simulink model "NavigationObserver_4"  (Simulink 8.3)
settings: configuration reference "mpc555rt_ref_debug_config" (kept outside this file)
values from neighbouring files (symbols this model uses):
  dt = 0.0192307692308    [newvars_4_25.mat]
  g = 32.174    [newvars_4_25.mat]
  P0_est_nav = [100 0 0 0 0 0 0 100 0 0 0 0 ... (36 elements, 6x6)]    [newvars_4_25.mat]
  Q_obs_nav = [0.001 0 0 0 0 0 0 0.001 0 0 0 0 ... (36 elements, 6x6)]    [newvars_4_25.mat]
  R_obs_nav = [0.001 0 0 0 0 0 0 0.001 0 0 0 0 ... (36 elements, 6x6)]    [newvars_4_25.mat]
  x0_est_nav = [0 0 200 0 0 0]    [newvars_4_25.mat]
libraries: simulink x1
(part 1 of 2)
settings Model: Creator=Rick Riley  LastModifiedBy=gagarcia
settings ConfigSet: SourceName=mpc555rt_ref_debug_config  SourceLocation=Base Workspace

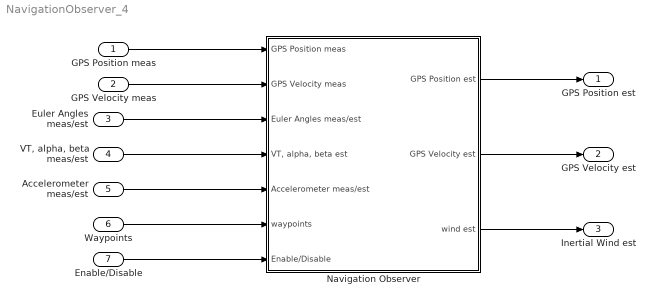
== system NavigationObserver_4 ==
  GPS Position meas : Inport  OutDataTypeStr=Bus: GPS_position_bus  SampleTime=dt
  GPS Velocity meas : Inport  Port=2  OutDataTypeStr=Bus: GPS_velocity_bus  SampleTime=dt  BusOutputAsStruct=on
  Euler Angles meas/est : Inport  Port=3  OutDataTypeStr=Bus: INS_angles_bus  SampleTime=dt
  "VT, alpha, beta meas/est" : Inport  Port=4  OutDataTypeStr=Bus: VT_A_B_bus  SampleTime=dt  BusOutputAsStruct=on
  Accelerometer meas/est : Inport  Port=5  OutDataTypeStr=Bus: Accelerometer
  Waypoints : Inport  Port=6  OutDataTypeStr=Bus: waypoint_bus  BusOutputAsStruct=on
  Enable/Disable : Inport  Port=7  OutDataTypeStr=boolean  SampleTime=dt
  Navigation Observer : Subsystem
  GPS Position est : Outport  OutDataTypeStr=Bus: GPS_position_bus  BusOutputAsStruct=on
  GPS Velocity est : Outport  Port=2  OutDataTypeStr=Bus: GPS_velocity_bus  BusOutputAsStruct=on
  Inertial Wind est : Outport  Port=3  OutDataTypeStr=Bus: Wind_bus  BusOutputAsStruct=on
  wires:
  Navigation Observer/3(wind est) -> Inertial Wind est/1
  GPS Position meas/1 -> Navigation Observer/1(GPS Position meas)
  GPS Velocity meas/1 -> Navigation Observer/2(GPS Velocity meas)
  Navigation Observer/1(GPS Position est) -> GPS Position est/1
  Navigation Observer/2(GPS Velocity est) -> GPS Velocity est/1
  Euler Angles meas/est/1 -> Navigation Observer/3(Euler Angles meas/est)
  "VT, alpha, beta meas/est"/1 -> Navigation Observer/4("VT, alpha, beta est")
  Accelerometer meas/est/1 -> Navigation Observer/5(Accelerometer meas/est)
  Waypoints/1 -> Navigation Observer/6(waypoints)
  Enable/Disable/1 -> Navigation Observer/7(Enable/Disable)

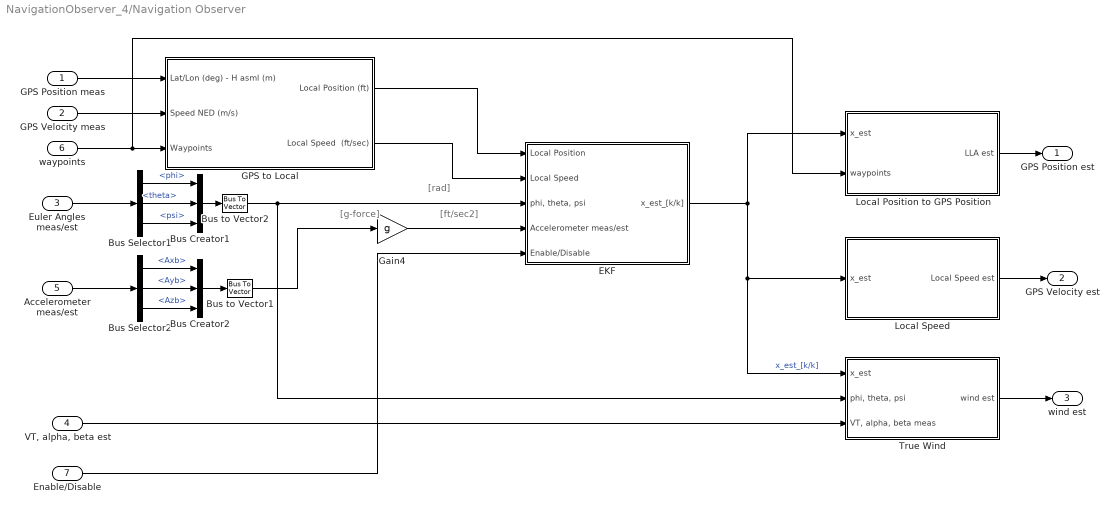
== system NavigationObserver_4/Navigation Observer ==
  note: [ft/sec2]
  note: [g-force]
  note: [rad]
  GPS Position meas : Inport  OutDataTypeStr=Bus: GPS_position_bus  SampleTime=dt
  GPS Velocity meas : Inport  Port=2  OutDataTypeStr=Bus: GPS_velocity_bus  SampleTime=dt  BusOutputAsStruct=on
  Euler Angles meas/est : Inport  Port=3  OutDataTypeStr=Bus: INS_angles_bus  SampleTime=dt
  "VT, alpha, beta est" : Inport  Port=4  OutDataTypeStr=Bus: VT_A_B_bus  SampleTime=dt  BusOutputAsStruct=on
  Accelerometer meas/est : Inport  Port=5  OutDataTypeStr=Bus: Accelerometer
  waypoints : Inport  Port=6  OutDataTypeStr=Bus: waypoint_bus
  Enable/Disable : Inport  Port=7  OutDataTypeStr=boolean  SampleTime=dt
  Bus Creator1 : BusCreator  Inputs=3  OutDataTypeStr=Bus: INS_angles_bus
  Bus Creator2 : BusCreator  Inputs=3  OutDataTypeStr=Bus: Accelerometer
  Bus Selector1 : BusSelector  OutputSignals=phi,theta,psi
  Bus Selector2 : BusSelector  OutputSignals=Axb,Ayb,Azb
  Bus to Vector1 : BusToVector
  Bus to Vector2 : BusToVector
  EKF : Subsystem
  GPS to Local : Subsystem
  Gain4 : Gain  Gain=g
  Local Position to GPS Position : Subsystem
  Local Speed : Subsystem
  True Wind : Subsystem
  GPS Position est : Outport  OutDataTypeStr=Bus: GPS_position_bus
  GPS Velocity est : Outport  Port=2
  wind est : Outport  Port=3
  wires:
  EKF/1(x_est_[k/k]) -> Local Position to GPS Position/1(x_est), Local Speed/1(x_est), True Wind/1(x_est)  "x_est_[k/k]"
  Euler Angles meas/est/1 -> Bus Selector1/1
  Accelerometer meas/est/1 -> Bus Selector2/1
  Bus to Vector1/1 -> Gain4/1
  GPS Position meas/1 -> GPS to Local/1(Lat/Lon (deg) - H asml (m))
  GPS Velocity meas/1 -> GPS to Local/2(Speed NED (m/s))
  waypoints/1 -> GPS to Local/3(Waypoints), Local Position to GPS Position/2(waypoints)
  GPS to Local/1(Local Position (ft)) -> EKF/1(Local Position)
  GPS to Local/2(Local Speed  (ft/sec)) -> EKF/2(Local Speed)
  Gain4/1 -> EKF/4(Accelerometer meas/est)
  Local Position to GPS Position/1(LLA est) -> GPS Position est/1
  Local Speed/1(Local Speed est) -> GPS Velocity est/1
  "VT, alpha, beta est"/1 -> True Wind/3("VT, alpha, beta meas")
  True Wind/1(wind est) -> wind est/1
  Bus to Vector2/1 -> EKF/3("phi, theta, psi"), True Wind/2("phi, theta, psi")
  Bus Selector1/1 -> Bus Creator1/1  "<phi>"
  Bus Selector1/2 -> Bus Creator1/2  "<theta>"
  Bus Selector1/3 -> Bus Creator1/3  "<psi>"
  Bus Creator1/1 -> Bus to Vector2/1
  Bus Selector2/1 -> Bus Creator2/1  "<Axb>"
  Bus Selector2/2 -> Bus Creator2/2  "<Ayb>"
  Bus Selector2/3 -> Bus Creator2/3  "<Azb>"
  Bus Creator2/1 -> Bus to Vector1/1
  Enable/Disable/1 -> EKF/5(Enable/Disable)

== system NavigationObserver_4/Navigation Observer/EKF ==
  Local Position : Inport
  Local Speed : Inport  Port=2
  "phi, theta, psi" : Inport  Port=3
  Accelerometer meas/est : Inport  Port=4
  Enable/Disable : Inport  Port=5  OutDataTypeStr=boolean  SampleTime=dt
  GPS rate correction : Subsystem
  Gain : Gain
  K[k] (navigation) : Subsystem
  Mux3 : Mux  Inputs=2
  Product : Product  RndMeth=Zero
  Product1 : Product  Multiplication=Matrix(*)  RndMeth=Zero
  Reshape1 : Reshape  OutputDimensionality=Column vector (2-D)
  Reshape2 : Reshape  OutputDimensionality=Column vector (2-D)
  Reshape3 : Reshape
  Subtract : Sum  Inputs=+-
  Subtract1 : Sum
  Unit Delay1 : UnitDelay  SampleTime=dt
  x_est_[0/0] : UnitDelay  InitialCondition=x0_est_nav  SampleTime=dt
  x_est_[k/k-1] : Subsystem
  y_[k] : Subsystem
  y_est_[k] : Subsystem
  x_est_[k/k] : Outport
  wires:
  y_[k]/1(y_[k]) -> Subtract/1, GPS rate correction/1(y_[k])
  Local Position/1 -> y_[k]/1(Local Position)
  x_est_[k/k-1]/1(x_est_[k/k-1]) -> y_est_[k]/1(x_est [k]), Reshape1/1
  Subtract1/1 -> Reshape3/1  "x_est_[k/k]"
  x_est_[0/0]/1 -> K[k] (navigation)/2(x_est_[k-1/k-1]), x_est_[k/k-1]/2(x_est_[k-1/k-1])  "x_est_[k-1/k-1]"
  Mux3/1 -> Unit Delay1/1  "u_[k]"
  Unit Delay1/1 -> K[k] (navigation)/1(u_[k-1]), x_est_[k/k-1]/1(u_[k-1])  "u_[k-1]"
  y_est_[k]/1(y_est_ [k]) -> Subtract/2
  Gain/1 -> Subtract1/1
  "phi, theta, psi"/1 -> Mux3/1
  Accelerometer meas/est/1 -> Mux3/2
  Local Speed/1 -> y_[k]/2(Local Speed)
  Product/1 -> Product1/1  "K_[k]"
  Product1/1 -> Gain/1
  Reshape1/1 -> Subtract1/2
  Reshape2/1 -> Product1/2
  Reshape3/1 -> x_est_[k/k]/1, x_est_[0/0]/1
  GPS rate correction/1(e_corrected_[k]) -> Reshape2/1
  Subtract/1 -> GPS rate correction/2(e_[k])
  K[k] (navigation)/1(K[k]) -> Product/1
  Enable/Disable/1 -> Product/2

== system NavigationObserver_4/Navigation Observer/GPS to Local ==
  Lat/Lon (deg) - H asml (m) : Inport
  Speed NED (m/s) : Inport  Port=2
  Waypoints : Inport  Port=3  OutDataTypeStr=Bus: waypoint_bus
  Bus Creator : BusCreator  Inputs=3  NonVirtualBus=on
  Bus Creator1 : BusCreator  Inputs=3  NonVirtualBus=on
  Bus Selector : BusSelector  OutputSignals=Altitude,Latitude,Longitude
  Bus Selector1 : BusSelector  OutputSignals=V_down,V_north,V_east
  Convert Lat/Lon/Alt to Flat Earth : MATLAB Function  TreatAsAtomicUnit=on
  Gain1 : Gain  Gain=-1
  Gain2 : Gain  Gain=1/.3048
  Gain3 : Gain  Gain=1/.3048
  Gain4 : Gain  Gain=1/.3048
  Local Position (ft) : Outport
  Local Speed  (ft/sec) : Outport  Port=2
  wires:
  Speed NED (m/s)/1 -> Bus Selector1/1
  Lat/Lon (deg) - H asml (m)/1 -> Bus Selector/1
  Bus Creator/1 -> Local Position (ft)/1
  Bus Selector1/2 -> Gain3/1  "<V_north>"
  Bus Selector1/1 -> Gain1/1  "<V_down>"
  Bus Selector1/3 -> Gain4/1  "<V_east>"
  Gain1/1 -> Gain2/1
  Gain4/1 -> Bus Creator1/3  "V_east"
  Gain3/1 -> Bus Creator1/2  "V_north"
  Gain2/1 -> Bus Creator1/1  "V_height"
  Bus Creator1/1 -> Local Speed  (ft/sec)/1
  Bus Selector/1 -> Convert Lat/Lon/Alt to Flat Earth/2(alt)  "<Altitude>"
  Bus Selector/2 -> Convert Lat/Lon/Alt to Flat Earth/3(lat)  "<Latitude>"
  Bus Selector/3 -> Convert Lat/Lon/Alt to Flat Earth/4(lon)  "<Longitude>"
  Convert Lat/Lon/Alt to Flat Earth/1(Height) -> Bus Creator/1
  Convert Lat/Lon/Alt to Flat Earth/2(North) -> Bus Creator/2
  Convert Lat/Lon/Alt to Flat Earth/3(East) -> Bus Creator/3
  Waypoints/1 -> Convert Lat/Lon/Alt to Flat Earth/1(wpts)

== system NavigationObserver_4/Navigation Observer/Local Position to GPS Position ==
  note: pn [ft]
  note: pe [ft]
  note: ph [ft]
  note: ve [ft/sec]
  note: vh [ft/sec]
  note: vn [ft/sec]
  x_est : Inport
  waypoints : Inport  Port=2  OutDataTypeStr=Bus: waypoint_bus
  Bus Creator : BusCreator  Inputs=3  OutDataTypeStr=Bus: GPS_position_bus  NonVirtualBus=on
  Convert Local Coordinates to LLA : MATLAB Function  TreatAsAtomicUnit=on
  Demux : Demux  Outputs=6
  Terminator : Terminator
  Terminator1 : Terminator
  Terminator2 : Terminator
  LLA est : Outport  OutDataTypeStr=Bus: GPS_position_bus
  wires:
  Convert Local Coordinates to LLA/3(Altitude) -> Bus Creator/3  "Altitude"
  Convert Local Coordinates to LLA/2(Longitude) -> Bus Creator/2  "Longitude"
  Convert Local Coordinates to LLA/1(Latitude) -> Bus Creator/1  "Latitude"
  x_est/1 -> Demux/1
  Bus Creator/1 -> LLA est/1
  Demux/4 -> Terminator/1
  Demux/5 -> Terminator1/1
  Demux/6 -> Terminator2/1
  Demux/1 -> Convert Local Coordinates to LLA/1(n)
  Demux/2 -> Convert Local Coordinates to LLA/2(e)
  Demux/3 -> Convert Local Coordinates to LLA/3(h)
  waypoints/1 -> Convert Local Coordinates to LLA/4(wpts)

== system NavigationObserver_4/Navigation Observer/Local Speed ==
  note: pn [ft]
  note: pe [ft]
  note: ph [ft]
  note: ve [ft/sec]
  note: vh [ft/sec]
  note: vn [ft/sec]
  x_est : Inport
  Bus Creator : BusCreator  Inputs=3  OutDataTypeStr=Bus: GPS_velocity_bus  NonVirtualBus=on
  Demux1 : Demux  Outputs=6
  Gain1 : Gain  Gain=0.3048
  Gain2 : Gain  Gain=0.3048
  Gain3 : Gain  Gain=-0.3048
  Terminator : Terminator
  Terminator1 : Terminator
  Terminator2 : Terminator
  Local Speed est : Outport
  wires:
  Bus Creator/1 -> Local Speed est/1
  Demux1/1 -> Terminator/1
  Demux1/2 -> Terminator1/1
  Demux1/3 -> Terminator2/1
  x_est/1 -> Demux1/1
  Gain2/1 -> Bus Creator/1  "V_north"
  Gain1/1 -> Bus Creator/2  "V_east"
  Gain3/1 -> Bus Creator/3  "V_down"
  Demux1/4 -> Gain2/1
  Demux1/5 -> Gain1/1
  Demux1/6 -> Gain3/1

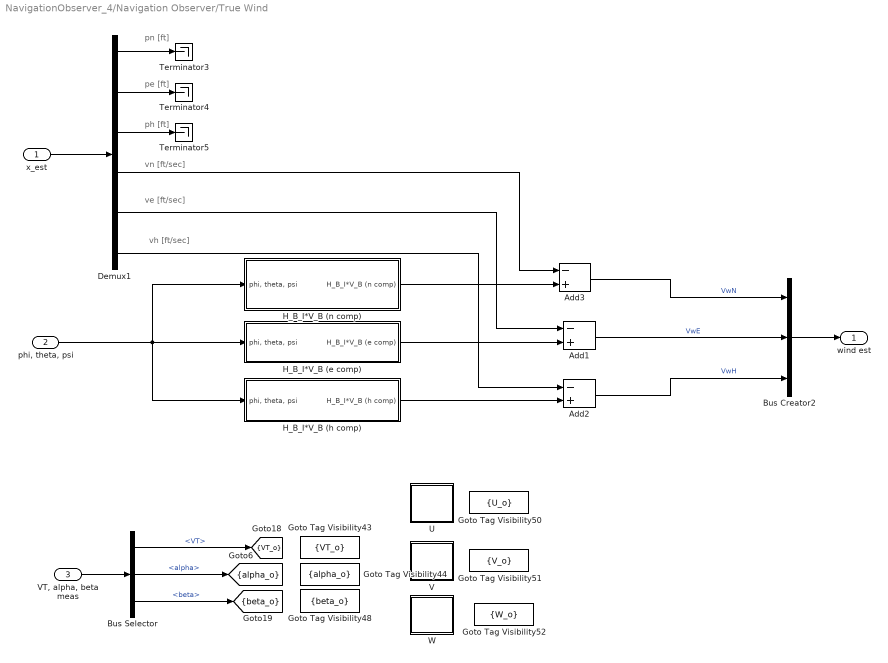
== system NavigationObserver_4/Navigation Observer/True Wind ==
  note: pn [ft]
  note: pe [ft]
  note: ph [ft]
  note: ve [ft/sec]
  note: vh [ft/sec]
  note: vn [ft/sec]
  x_est : Inport
  "phi, theta, psi" : Inport  Port=2
  "VT, alpha, beta meas" : Inport  Port=3
  Add1 : Sum  Inputs=-+
  Add2 : Sum  Inputs=-+
  Add3 : Sum  Inputs=-+
  Bus Creator2 : BusCreator  Inputs=3  OutDataTypeStr=Bus: Wind_bus  NonVirtualBus=on
  Bus Selector : BusSelector  OutputSignals=VT,alpha,beta
  Demux1 : Demux  Outputs=6
  Goto Tag Visibility43 : GotoTagVisibility  GotoTag=VT_o
  Goto Tag Visibility44 : GotoTagVisibility  GotoTag=alpha_o
  Goto Tag Visibility48 : GotoTagVisibility  GotoTag=beta_o
  Goto Tag Visibility50 : GotoTagVisibility  GotoTag=U_o
  Goto Tag Visibility51 : GotoTagVisibility  GotoTag=V_o
  Goto Tag Visibility52 : GotoTagVisibility  GotoTag=W_o
  H_B_I*V_B (e comp) : Subsystem
  H_B_I*V_B (h comp) : Subsystem
  H_B_I*V_B (n comp) : Subsystem
  Terminator3 : Terminator
  Terminator4 : Terminator
  Terminator5 : Terminator
  U : Subsystem
  V : Subsystem
  W : Subsystem
  wind est : Outport
  tag scope: VT_o=scoped, alpha_o=scoped, beta_o=scoped
  wires:
  "phi, theta, psi"/1 -> H_B_I*V_B (n comp)/1("phi, theta, psi"), H_B_I*V_B (e comp)/1("phi, theta, psi"), H_B_I*V_B (h comp)/1("phi, theta, psi")
  "VT, alpha, beta meas"/1 -> Bus Selector/1
  Demux1/1 -> Terminator3/1
  Demux1/2 -> Terminator4/1
  Demux1/3 -> Terminator5/1
  x_est/1 -> Demux1/1
  Demux1/4 -> Add3/1
  Demux1/5 -> Add1/1
  Demux1/6 -> Add2/1
  Bus Selector/1 -> [VT_o]  "<VT>"
  Bus Selector/2 -> [alpha_o]  "<alpha>"
  Bus Selector/3 -> [beta_o]  "<beta>"
  Add3/1 -> Bus Creator2/1  "VwN"
  Add1/1 -> Bus Creator2/2  "VwE"
  Add2/1 -> Bus Creator2/3  "VwH"
  Bus Creator2/1 -> wind est/1
  H_B_I*V_B (n comp)/1(H_B_I*V_B (n comp)) -> Add3/2
  H_B_I*V_B (e comp)/1(H_B_I*V_B (e comp)) -> Add1/2
  H_B_I*V_B (h comp)/1(H_B_I*V_B (h comp)) -> Add2/2

== system NavigationObserver_4/Navigation Observer/EKF/GPS rate correction ==
  note: e_pn [ft]
  note: e_pe [ft]
  note: e_ph [ft]
  note: e_vn [ft/sec]
  note: e_ve [ft/sec]
  note: e_vh [ft/sec]
  y_[k] : Inport
  e_[k] : Inport  Port=2
  Constant : Constant  Value=0
  Demux1 : Demux  Outputs=6
  Detect Change : simulink/Logic and Bit Operations/Detect Change  vinit=0  InputProcessing=Inherited  OutDataTypeStr=uint8
  Mux : Mux  Inputs=6
  Selector : Selector  InputPortWidth=6  Indices=[1]
  Switch{,1..5} (6 alike) : Switch  Criteria=u2 > Threshold
  e_corrected_[k] : Outport
  wires:
  Mux/1 -> e_corrected_[k]/1
  e_[k]/1 -> Demux1/1
  Demux1/1 -> Switch/1
  Switch/1 -> Mux/1
  Selector/1 -> Detect Change/1
  y_[k]/1 -> Selector/1
  Demux1/3 -> Switch2/1
  Demux1/2 -> Switch1/1
  Demux1/4 -> Switch3/1
  Demux1/5 -> Switch4/1
  Demux1/6 -> Switch5/1
  Switch1/1 -> Mux/2
  Switch2/1 -> Mux/3
  Switch3/1 -> Mux/4
  Switch4/1 -> Mux/5
  Switch5/1 -> Mux/6
  Constant/1 -> Switch/3, Switch1/3, Switch2/3, Switch3/3, Switch4/3, Switch5/3
  Detect Change/1 -> Switch/2, Switch1/2, Switch2/2, Switch3/2, Switch4/2, Switch5/2

== system NavigationObserver_4/Navigation Observer/EKF/K[k] (navigation) ==
  u_[k-1] : Inport
  x_est_[k-1/k-1] : Inport  Port=2
  H_[k] : Constant  Value=eye(6)
  Jacobian F : Subsystem
  K_[k] : Subsystem
  P_est_[0/0] : UnitDelay  InitialCondition=P0_est_nav  SampleTime=dt
  Product1 : Product  Inputs=3  Multiplication=Matrix(*)  RndMeth=Zero
  Product3 : Product  Inputs=3  Multiplication=Matrix(*)  RndMeth=Zero
  Q_[k-1] : Constant  Value=Q_obs_nav
  R_[k] : Constant  Value=R_obs_nav
  Subtract1 : Sum
  Subtract4 : Sum  Inputs=+-
  Transpose : MATLAB Function  TreatAsAtomicUnit=on
  K[k] : Outport
  wires:
  x_est_[k-1/k-1]/1 -> Jacobian F/2(x_est_[k-1/k-1])
  u_[k-1]/1 -> Jacobian F/1(u_[k-1])
  Jacobian F/1(F_[k-1]) -> Transpose/1(u), Product1/1  "F_[k-1]"
  P_est_[0/0]/1 -> Product1/2  "P_[k-1/k-1]"
  Subtract4/1 -> P_est_[0/0]/1  "P_[k/k]"
  Product3/1 -> Subtract4/2
  K_[k]/1(K_[k]) -> K[k]/1, Product3/1  "K_[k]"
  R_[k]/1 -> K_[k]/2(R_[k])  "R_[k]"
  H_[k]/1 -> K_[k]/3(H_[k]), Product3/2  "H_[k]"
  Subtract1/1 -> Product3/3, Subtract4/1, K_[k]/1(P_[k/k-1])  "P_[k/k-1]"
  Q_[k-1]/1 -> Subtract1/2  "Q_[k-1]"
  Product1/1 -> Subtract1/1  "F_{k-1] P_[k-1/k-1] F'_[k-1]"
  Transpose/1(FT_k_1) -> Product1/3  "FT_k_1"

== system NavigationObserver_4/Navigation Observer/EKF/x_est_[k/k-1] ==
  u_[k-1] : Inport
  x_est_[k-1/k-1] : Inport  Port=2
  Gain4 : Gain  Gain=dt
  Subtract1 : Sum
  f(x_est_[k],u_[k]) : Subsystem
  x_est_[k/k-1] : Outport
  wires:
  f(x_est_[k],u_[k])/1(f_(x_est_[k],u_[k])) -> Gain4/1
  Gain4/1 -> Subtract1/2
  x_est_[k-1/k-1]/1 -> Subtract1/1, f(x_est_[k],u_[k])/1(x_est [k])
  u_[k-1]/1 -> f(x_est_[k],u_[k])/2(u_[k])
  Subtract1/1 -> x_est_[k/k-1]/1

== system NavigationObserver_4/Navigation Observer/EKF/y_[k] ==
  note: pn [ft]
  note: pe [ft]
  note: ph [ft]
  note: ve [ft/sec]
  note: vh [ft/sec]
  note: vn [ft/sec]
  Local Position : Inport
  Local Speed : Inport  Port=2
  Bus Selector2 : BusSelector  OutputSignals=North,East,Height
  Bus Selector3 : BusSelector  OutputSignals=V_north,V_east,V_height
  Mux : Mux  Inputs=6
  y_[k] : Outport
  wires:
  Mux/1 -> y_[k]/1
  Local Position/1 -> Bus Selector2/1
  Local Speed/1 -> Bus Selector3/1
  Bus Selector2/1 -> Mux/1  "<North>"
  Bus Selector2/2 -> Mux/2  "<East>"
  Bus Selector2/3 -> Mux/3  "<Height>"
  Bus Selector3/1 -> Mux/4  "<V_north>"
  Bus Selector3/2 -> Mux/5  "<V_east>"
  Bus Selector3/3 -> Mux/6  "<V_height>"

== system NavigationObserver_4/Navigation Observer/EKF/y_est_[k] ==
  x_est [k] : Inport
  h(x_est_[k],u_[k]) : Subsystem
  y_est_ [k] : Outport
  wires:
  x_est [k]/1 -> h(x_est_[k],u_[k])/1(x_est [k])
  h(x_est_[k],u_[k])/1(y_est_ [k]) -> y_est_ [k]/1

== system NavigationObserver_4/Navigation Observer/True Wind/H_B_I*V_B (e comp) ==
  note: theta [rad]
  note: phi [rad]
  note: psi [rad]
  note: U [ft/sec]
  note: V [ft/sec]
  note: W [ft/sec]
  "phi, theta, psi" : Inport
  Add1 : Sum
  Add2 : Sum  Inputs=+++
  Add3 : Sum  Inputs=-+
  Demux2 : Demux  Outputs=3
  Divide{1,4,6..7} (4 alike) : Product  Inputs=**
  Divide2 : Product  Inputs=***
  Divide3 : Product  Inputs=***
  Divide5 : Product  Inputs=***
  Trigonometric Function : Trigonometry
  Trigonometric Function1 : Trigonometry  Operator=cos
  Trigonometric Function2 : Trigonometry
  Trigonometric Function3 : Trigonometry
  Trigonometric Function4 : Trigonometry  Operator=cos
  Trigonometric Function5 : Trigonometry  Operator=cos
  H_B_I*V_B (e comp) : Outport
  wires:
  Demux2/3 -> Trigonometric Function3/1, Trigonometric Function4/1
  Demux2/2 -> Trigonometric Function2/1, Trigonometric Function1/1
  Demux2/1 -> Trigonometric Function/1, Trigonometric Function5/1
  [V_o] -> Divide1/2
  [W_o] -> Divide7/2
  Trigonometric Function/1 -> Divide6/1, Divide2/2
  Trigonometric Function2/1 -> Divide5/1, Divide2/1
  Trigonometric Function4/1 -> Divide6/2, Divide4/2
  Trigonometric Function5/1 -> Divide5/2, Divide4/1
  Trigonometric Function3/1 -> Divide3/3, Divide5/3, Divide2/3
  Divide7/1 -> Add2/3
  Add3/1 -> Divide7/1
  Divide5/1 -> Add3/2
  Divide6/1 -> Add3/1
  Divide1/1 -> Add2/2
  Divide3/1 -> Add2/1
  Divide2/1 -> Add1/2
  Divide4/1 -> Add1/1
  Add1/1 -> Divide1/1
  Trigonometric Function1/1 -> Divide3/2
  [U_o] -> Divide3/1
  Add2/1 -> H_B_I*V_B (e comp)/1
  "phi, theta, psi"/1 -> Demux2/1

== system NavigationObserver_4/Navigation Observer/True Wind/H_B_I*V_B (h comp) ==
  note: theta [rad]
  note: phi [rad]
  note: U [ft/sec]
  note: V [ft/sec]
  note: W [ft/sec]
  "phi, theta, psi" : Inport
  Add1 : Sum  Inputs=+--
  Demux2 : Demux  Outputs=3
  Divide1 : Product  Inputs=***
  Divide2 : Product  Inputs=**
  Divide3 : Product  Inputs=***
  Terminator2 : Terminator
  Trigonometric Function : Trigonometry
  Trigonometric Function1 : Trigonometry  Operator=cos
  Trigonometric Function2 : Trigonometry
  Trigonometric Function4 : Trigonometry  Operator=cos
  Trigonometric Function5 : Trigonometry  Operator=cos
  H_B_I*V_B (h comp) : Outport
  wires:
  Demux2/1 -> Trigonometric Function4/1, Trigonometric Function2/1
  Demux2/2 -> Trigonometric Function5/1, Trigonometric Function1/1, Trigonometric Function/1
  Divide1/1 -> Add1/3
  [W_o] -> Divide1/3
  Trigonometric Function5/1 -> Divide1/2
  Trigonometric Function4/1 -> Divide1/1
  Divide2/1 -> Add1/1
  Divide3/1 -> Add1/2
  [V_o] -> Divide3/3
  Trigonometric Function2/1 -> Divide3/2
  Trigonometric Function1/1 -> Divide3/1
  Trigonometric Function/1 -> Divide2/2
  [U_o] -> Divide2/1
  "phi, theta, psi"/1 -> Demux2/1
  Demux2/3 -> Terminator2/1
  Add1/1 -> H_B_I*V_B (h comp)/1

== system NavigationObserver_4/Navigation Observer/True Wind/H_B_I*V_B (n comp) ==
  note: U [ft/sec]
  note: V [ft/sec]
  note: W [ft/sec]
  note: theta [rad]
  note: phi [rad]
  note: psi [rad]
  "phi, theta, psi" : Inport
  Add1 : Sum  Inputs=-+
  Add2 : Sum  Inputs=+++
  Add3 : Sum
  Demux2 : Demux  Outputs=3
  Divide{1,4,6..7} (4 alike) : Product  Inputs=**
  Divide2 : Product  Inputs=***
  Divide3 : Product  Inputs=***
  Divide5 : Product  Inputs=***
  Trigonometric Function : Trigonometry
  Trigonometric Function1 : Trigonometry  Operator=cos
  Trigonometric Function2 : Trigonometry
  Trigonometric Function3 : Trigonometry
  Trigonometric Function4 : Trigonometry  Operator=cos
  Trigonometric Function5 : Trigonometry  Operator=cos
  H_B_I*V_B (n comp) : Outport
  wires:
  "phi, theta, psi"/1 -> Demux2/1
  Divide7/1 -> Add2/3
  Add3/1 -> Divide7/1
  Divide5/1 -> Add3/2
  Divide6/1 -> Add3/1
  Divide1/1 -> Add2/2
  Divide3/1 -> Add2/1
  Trigonometric Function/1 -> Divide6/1, Divide2/2
  Trigonometric Function2/1 -> Divide5/1, Divide2/1
  Trigonometric Function3/1 -> Divide6/2, Divide4/2
  Trigonometric Function5/1 -> Divide5/2, Divide4/1
  Divide2/1 -> Add1/2
  Divide4/1 -> Add1/1
  Add1/1 -> Divide1/1
  Trigonometric Function4/1 -> Divide5/3, Divide2/3, Divide3/3
  Trigonometric Function1/1 -> Divide3/2
  Demux2/3 -> Trigonometric Function3/1, Trigonometric Function4/1
  Demux2/1 -> Trigonometric Function/1, Trigonometric Function5/1
  Demux2/2 -> Trigonometric Function2/1, Trigonometric Function1/1
  Add2/1 -> H_B_I*V_B (n comp)/1
  [W_o] -> Divide7/2
  [V_o] -> Divide1/2
  [U_o] -> Divide3/1

== system NavigationObserver_4/Navigation Observer/True Wind/U ==
  Divide2 : Product  Inputs=***
  Trigonometric Function : Trigonometry  Operator=cos
  Trigonometric Function1 : Trigonometry  Operator=cos
  tag scope: U_o=scoped
  wires:
  [beta_o] -> Trigonometric Function1/1
  [alpha_o] -> Trigonometric Function/1
  Trigonometric Function1/1 -> Divide2/3
  Trigonometric Function/1 -> Divide2/2
  [VT_o] -> Divide2/1
  Divide2/1 -> [U_o]

== system NavigationObserver_4/Navigation Observer/True Wind/V ==
  Divide2 : Product  Inputs=**
  Trigonometric Function1 : Trigonometry
  tag scope: V_o=scoped
  wires:
  [beta_o] -> Trigonometric Function1/1
  Trigonometric Function1/1 -> Divide2/2
  [VT_o] -> Divide2/1
  Divide2/1 -> [V_o]

== system NavigationObserver_4/Navigation Observer/True Wind/W ==
  Divide2 : Product  Inputs=***
  Trigonometric Function : Trigonometry
  Trigonometric Function1 : Trigonometry  Operator=cos
  tag scope: W_o=scoped
  wires:
  [beta_o] -> Trigonometric Function1/1
  [alpha_o] -> Trigonometric Function/1
  Trigonometric Function1/1 -> Divide2/3
  Trigonometric Function/1 -> Divide2/2
  [VT_o] -> Divide2/1
  Divide2/1 -> [W_o]

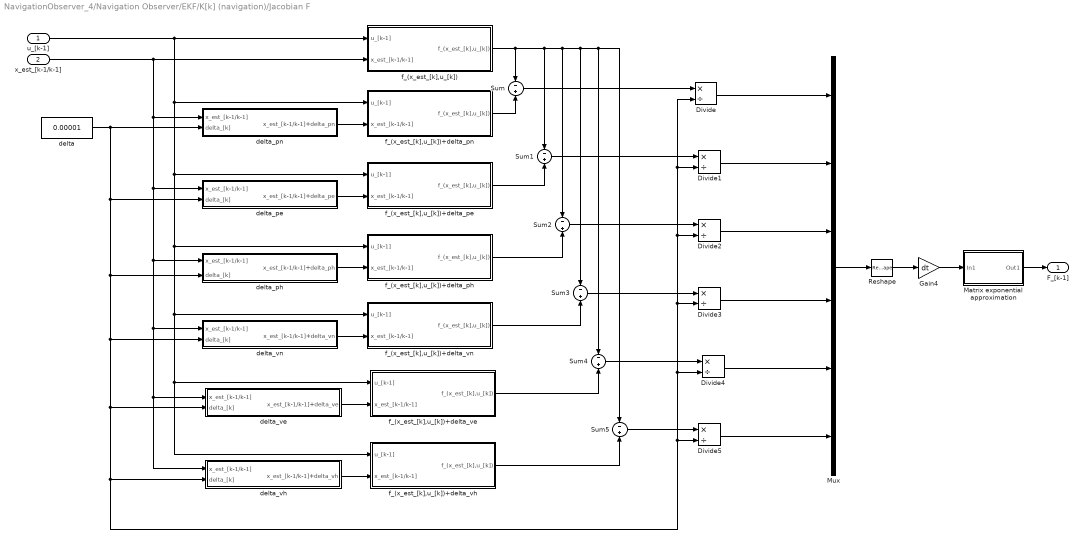
== system NavigationObserver_4/Navigation Observer/EKF/K[k] (navigation)/Jacobian F ==
  u_[k-1] : Inport
  x_est_[k-1/k-1] : Inport  Port=2
  Divide{,1..5} (6 alike) : Product  Inputs=*/
  Gain4 : Gain  Gain=dt
  Matrix exponential approximation : Subsystem
  Mux : Mux  Inputs=6
  Reshape : Reshape  OutputDimensionality=Customize  OutputDimensions=[6,6]
  Sum{,1..5} (6 alike) : Sum  Inputs=-|+
  delta : Constant  Value=0.00001
  delta_pe : Subsystem
  delta_ph : Subsystem
  delta_pn : Subsystem
  delta_ve : Subsystem
  delta_vh : Subsystem
  delta_vn : Subsystem
  f_(x_est_[k],u_[k]) : Subsystem
  f_(x_est_[k],u_[k])+delta_pe : Subsystem
  f_(x_est_[k],u_[k])+delta_ph : Subsystem
  f_(x_est_[k],u_[k])+delta_pn : Subsystem
  f_(x_est_[k],u_[k])+delta_ve : Subsystem
  f_(x_est_[k],u_[k])+delta_vh : Subsystem
  f_(x_est_[k],u_[k])+delta_vn : Subsystem
  F_[k-1] : Outport
  wires:
  Gain4/1 -> Matrix exponential approximation/1(In1)
  Matrix exponential approximation/1(Out1) -> F_[k-1]/1
  Mux/1 -> Reshape/1
  delta/1 -> delta_pn/2(delta_[k]), delta_pe/2(delta_[k]), delta_vn/2(delta_[k]), delta_ve/2(delta_[k]), Divide5/2, Divide4/2, Divide3/2, Divide2/2, Divide1/2, Divide/2, delta_vh/2(delta_[k]), delta_ph/2(delta_[k])
  delta_pn/1(x_est_[k-1/k-1]+delta_pn) -> f_(x_est_[k],u_[k])+delta_pn/2(x_est_[k-1/k-1])
  f_(x_est_[k],u_[k])/1(f_(x_est_[k],u_[k])) -> Sum/1, Sum1/1, Sum2/1, Sum3/1, Sum5/1, Sum4/1
  f_(x_est_[k],u_[k])+delta_pn/1(f_(x_est_[k],u_[k])) -> Sum/2
  Sum/1 -> Divide/1
  u_[k-1]/1 -> f_(x_est_[k],u_[k])/1(u_[k-1]), f_(x_est_[k],u_[k])+delta_pn/1(u_[k-1]), f_(x_est_[k],u_[k])+delta_pe/1(u_[k-1]), f_(x_est_[k],u_[k])+delta_ph/1(u_[k-1]), f_(x_est_[k],u_[k])+delta_vn/1(u_[k-1]), f_(x_est_[k],u_[k])+delta_vh/1(u_[k-1]), f_(x_est_[k],u_[k])+delta_ve/1(u_[k-1])
  x_est_[k-1/k-1]/1 -> f_(x_est_[k],u_[k])/2(x_est_[k-1/k-1]), delta_pn/1(x_est_[k-1/k-1]), delta_pe/1(x_est_[k-1/k-1]), delta_ph/1(x_est_[k-1/k-1]), delta_vn/1(x_est_[k-1/k-1]), delta_vh/1(x_est_[k-1/k-1]), delta_ve/1(x_est_[k-1/k-1])
  delta_pe/1(x_est_[k-1/k-1]+delta_pe) -> f_(x_est_[k],u_[k])+delta_pe/2(x_est_[k-1/k-1])
  f_(x_est_[k],u_[k])+delta_pe/1(f_(x_est_[k],u_[k])) -> Sum1/2
  Sum1/1 -> Divide1/1
  delta_ph/1(x_est_[k-1/k-1]+delta_ph) -> f_(x_est_[k],u_[k])+delta_ph/2(x_est_[k-1/k-1])
  f_(x_est_[k],u_[k])+delta_ph/1(f_(x_est_[k],u_[k])) -> Sum2/2
  delta_vn/1(x_est_[k-1/k-1]+delta_vn) -> f_(x_est_[k],u_[k])+delta_vn/2(x_est_[k-1/k-1])
  f_(x_est_[k],u_[k])+delta_vn/1(f_(x_est_[k],u_[k])) -> Sum3/2
  Sum2/1 -> Divide2/1
  Sum3/1 -> Divide3/1
  delta_ve/1(x_est_[k-1/k-1]+delta_ve) -> f_(x_est_[k],u_[k])+delta_ve/2(x_est_[k-1/k-1])
  f_(x_est_[k],u_[k])+delta_ve/1(f_(x_est_[k],u_[k])) -> Sum4/2
  Sum4/1 -> Divide4/1
  delta_vh/1(x_est_[k-1/k-1]+delta_vh) -> f_(x_est_[k],u_[k])+delta_vh/2(x_est_[k-1/k-1])
  f_(x_est_[k],u_[k])+delta_vh/1(f_(x_est_[k],u_[k])) -> Sum5/2
  Sum5/1 -> Divide5/1
  Divide5/1 -> Mux/6
  Divide4/1 -> Mux/5
  Divide3/1 -> Mux/4
  Divide2/1 -> Mux/3
  Divide1/1 -> Mux/2
  Divide/1 -> Mux/1
  Reshape/1 -> Gain4/1

== system NavigationObserver_4/Navigation Observer/EKF/K[k] (navigation)/K_[k] ==
  P_[k/k-1] : Inport
  R_[k] : Inport  Port=2
  H_[k] : Inport  Port=3
  Inverse : MATLAB Function  TreatAsAtomicUnit=on
  Product : Product  Inputs=3  Multiplication=Matrix(*)  RndMeth=Zero
  Product1 : Product  Inputs=3  Multiplication=Matrix(*)  RndMeth=Zero
  Subtract2 : Sum
  Transpose : MATLAB Function  TreatAsAtomicUnit=on
  K_[k] : Outport
  wires:
  Inverse/1(y) -> Product1/3
  Product1/1 -> K_[k]/1
  Subtract2/1 -> Inverse/1(u)
  R_[k]/1 -> Subtract2/2
  Product/1 -> Subtract2/1
  Transpose/1(HT_k) -> Product/3, Product1/2  "HT_k"
  P_[k/k-1]/1 -> Product1/1, Product/2  "P_[k/k-1]"
  H_[k]/1 -> Transpose/1(u), Product/1  "H_[k]"

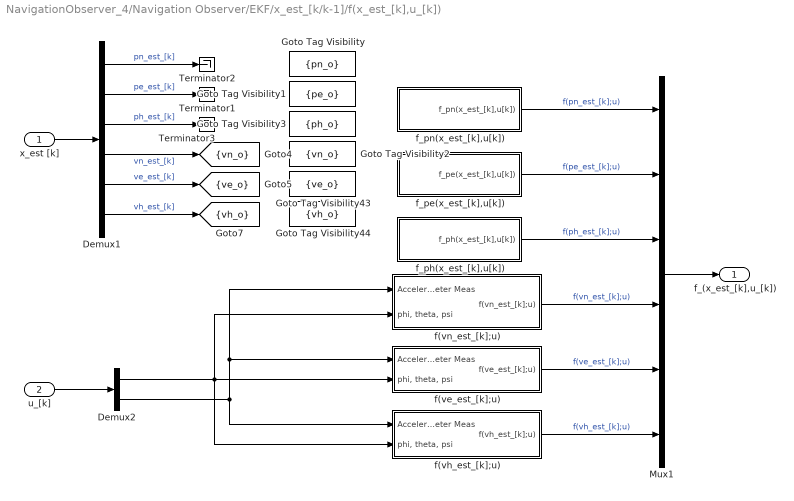
== system NavigationObserver_4/Navigation Observer/EKF/x_est_[k/k-1]/f(x_est_[k],u_[k]) ==
  x_est [k] : Inport
  u_[k] : Inport  Port=2
  Demux1 : Demux  Outputs=6
  Demux2 : Demux  Outputs=2
  Goto Tag Visibility : GotoTagVisibility  GotoTag=pn_o
  Goto Tag Visibility1 : GotoTagVisibility  GotoTag=pe_o
  Goto Tag Visibility2 : GotoTagVisibility  GotoTag=vn_o
  Goto Tag Visibility3 : GotoTagVisibility  GotoTag=ph_o
  Goto Tag Visibility43 : GotoTagVisibility  GotoTag=ve_o
  Goto Tag Visibility44 : GotoTagVisibility  GotoTag=vh_o
  Mux1 : Mux  Inputs=6
  Terminator1 : Terminator
  Terminator2 : Terminator
  Terminator3 : Terminator
  f(ve_est_[k];u) : Subsystem
  f(vh_est_[k];u) : Subsystem
  f(vn_est_[k];u) : Subsystem
  f_pe(x_est_[k],u[k]) : Subsystem
  f_ph(x_est_[k],u[k]) : Subsystem
  f_pn(x_est_[k],u[k]) : Subsystem
  f_(x_est_[k],u_[k]) : Outport
  tag scope: ve_o=scoped, vh_o=scoped, vn_o=scoped
  wires:
  Demux1/1 -> Terminator2/1  "pn_est_[k]"
  Demux1/2 -> Terminator1/1  "pe_est_[k]"
  Demux1/3 -> Terminator3/1  "ph_est_[k]"
  Demux1/4 -> [vn_o]  "vn_est_[k]"
  Demux1/6 -> [vh_o]  "vh_est_[k]"
  x_est [k]/1 -> Demux1/1
  Demux1/5 -> [ve_o]  "ve_est_[k]"
  f(vh_est_[k];u)/1(f(vh_est_[k];u)) -> Mux1/6  "f(vh_est_[k];u)"
  Mux1/1 -> f_(x_est_[k],u_[k])/1
  f(ve_est_[k];u)/1(f(ve_est_[k];u)) -> Mux1/5  "f(ve_est_[k];u)"
  f(vn_est_[k];u)/1(f(vn_est_[k];u)) -> Mux1/4  "f(vn_est_[k];u)"
  f_ph(x_est_[k],u[k])/1(f_ph(x_est_[k],u[k])) -> Mux1/3  "f(ph_est_[k];u)"
  f_pn(x_est_[k],u[k])/1(f_pn(x_est_[k],u[k])) -> Mux1/1  "f(pn_est_[k];u)"
  f_pe(x_est_[k],u[k])/1(f_pe(x_est_[k],u[k])) -> Mux1/2  "f(pe_est_[k];u)"
  u_[k]/1 -> Demux2/1
  Demux2/1 -> f(ve_est_[k];u)/2("phi, theta, psi"), f(vh_est_[k];u)/2("phi, theta, psi"), f(vn_est_[k];u)/2("phi, theta, psi")
  Demux2/2 -> f(vn_est_[k];u)/1(Accelerometer Meas), f(ve_est_[k];u)/1(Accelerometer Meas), f(vh_est_[k];u)/1(Accelerometer Meas)

== system NavigationObserver_4/Navigation Observer/EKF/y_est_[k]/h(x_est_[k],u_[k]) ==
  note: pn [ft]
  note: pe [ft]
  note: ph [ft]
  note: ve [ft/sec]
  note: vh [ft/sec]
  note: vn [ft/sec]
  x_est [k] : Inport
  Demux2 : Demux  Outputs=6
  Mux1 : Mux  Inputs=6
  y_est_ [k] : Outport
  wires:
  x_est [k]/1 -> Demux2/1
  Demux2/1 -> Mux1/1  "pn_est_[k]"
  Demux2/2 -> Mux1/2  "pe_est_[k]"
  Demux2/3 -> Mux1/3  "ph_est_[k]"
  Demux2/4 -> Mux1/4  "vn_est_[k]"
  Demux2/6 -> Mux1/6  "vh_est_[k]"
  Demux2/5 -> Mux1/5  "ve_est_[k]"
  Mux1/1 -> y_est_ [k]/1

== system NavigationObserver_4/Navigation Observer/EKF/K[k] (navigation)/Jacobian F/Matrix exponential approximation ==
  In1 : Inport
  Add : Sum  Inputs=+++++
  Constant : Constant  Value=eye(6)
  Gain : Gain  Gain=1/2
  Gain1 : Gain  Gain=1/6
  Gain2 : Gain  Gain=1/24
  Matrix Multiply : Product  Multiplication=Matrix(*)
  Matrix Multiply1 : Product  Multiplication=Matrix(*)
  Matrix Multiply2 : Product  Multiplication=Matrix(*)
  Out1 : Outport
  wires:
  Gain2/1 -> Add/5
  Matrix Multiply2/1 -> Gain2/1
  Gain1/1 -> Add/4
  Matrix Multiply1/1 -> Matrix Multiply2/1, Gain1/1
  Add/1 -> Out1/1
  Constant/1 -> Add/1
  Gain/1 -> Add/3
  Matrix Multiply/1 -> Matrix Multiply1/1, Gain/1
  In1/1 -> Matrix Multiply/1, Add/2, Matrix Multiply/2, Matrix Multiply2/2, Matrix Multiply1/2

== system NavigationObserver_4/Navigation Observer/EKF/K[k] (navigation)/Jacobian F/delta_pe ==
  x_est_[k-1/k-1] : Inport
  delta_[k] : Inport  Port=2
  Add1 : Sum
  Demux2 : Demux  Outputs=6
  Mux1 : Mux  Inputs=6
  x_est_[k-1/k-1]+delta_pe : Outport
  wires:
  Add1/1 -> Mux1/2
  Demux2/1 -> Mux1/1  "pn_est_[k]"
  Mux1/1 -> x_est_[k-1/k-1]+delta_pe/1
  Demux2/2 -> Add1/2  "pe_est_[k]"
  Demux2/3 -> Mux1/3  "ph_est_[k]"
  Demux2/4 -> Mux1/4  "vn_est_[k]"
  Demux2/6 -> Mux1/6  "vh_est_[k]"
  Demux2/5 -> Mux1/5  "ve_est_[k]"
  x_est_[k-1/k-1]/1 -> Demux2/1
  delta_[k]/1 -> Add1/1

== system NavigationObserver_4/Navigation Observer/EKF/K[k] (navigation)/Jacobian F/delta_ph ==
  x_est_[k-1/k-1] : Inport
  delta_[k] : Inport  Port=2
  Add : Sum
  Demux2 : Demux  Outputs=6
  Mux1 : Mux  Inputs=6
  x_est_[k-1/k-1]+delta_ph : Outport
  wires:
  Demux2/1 -> Mux1/1  "pn_est_[k]"
  Add/1 -> Mux1/3
  Mux1/1 -> x_est_[k-1/k-1]+delta_ph/1
  Demux2/2 -> Mux1/2  "pe_est_[k]"
  Demux2/3 -> Add/2  "ph_est_[k]"
  Demux2/4 -> Mux1/4  "vn_est_[k]"
  Demux2/6 -> Mux1/6  "vh_est_[k]"
  Demux2/5 -> Mux1/5  "ve_est_[k]"
  x_est_[k-1/k-1]/1 -> Demux2/1
  delta_[k]/1 -> Add/1

== system NavigationObserver_4/Navigation Observer/EKF/K[k] (navigation)/Jacobian F/delta_pn ==
  x_est_[k-1/k-1] : Inport
  delta_[k] : Inport  Port=2
  Add : Sum
  Demux1 : Demux  Outputs=6
  Mux : Mux  Inputs=6
  x_est_[k-1/k-1]+delta_pn : Outport
  wires:
  Mux/1 -> x_est_[k-1/k-1]+delta_pn/1
  Add/1 -> Mux/1
  Demux1/1 -> Add/2  "pn_est_[k]"
  Demux1/2 -> Mux/2  "pe_est_[k]"
  Demux1/3 -> Mux/3  "ph_est_[k]"
  Demux1/4 -> Mux/4  "vn_est_[k]"
  Demux1/6 -> Mux/6  "vh_est_[k]"
  Demux1/5 -> Mux/5  "ve_est_[k]"
  x_est_[k-1/k-1]/1 -> Demux1/1
  delta_[k]/1 -> Add/1

== system NavigationObserver_4/Navigation Observer/EKF/K[k] (navigation)/Jacobian F/delta_ve ==
  x_est_[k-1/k-1] : Inport
  delta_[k] : Inport  Port=2
  Add : Sum
  Demux2 : Demux  Outputs=6
  Mux1 : Mux  Inputs=6
  x_est_[k-1/k-1]+delta_ve : Outport
  wires:
  Add/1 -> Mux1/5
  Mux1/1 -> x_est_[k-1/k-1]+delta_ve/1
  Demux2/1 -> Mux1/1  "pn_est_[k]"
  Demux2/2 -> Mux1/2  "pe_est_[k]"
  Demux2/3 -> Mux1/3  "ph_est_[k]"
  Demux2/4 -> Mux1/4  "vn_est_[k]"
  Demux2/6 -> Mux1/6  "vh_est_[k]"
  Demux2/5 -> Add/2  "ve_est_[k]"
  x_est_[k-1/k-1]/1 -> Demux2/1
  delta_[k]/1 -> Add/1

== system NavigationObserver_4/Navigation Observer/EKF/K[k] (navigation)/Jacobian F/delta_vh ==
  x_est_[k-1/k-1] : Inport
  delta_[k] : Inport  Port=2
  Add1 : Sum
  Demux2 : Demux  Outputs=6
  Mux1 : Mux  Inputs=6
  x_est_[k-1/k-1]+delta_vh : Outport
  wires:
  Add1/1 -> Mux1/6
  Mux1/1 -> x_est_[k-1/k-1]+delta_vh/1
  Demux2/1 -> Mux1/1  "pn_est_[k]"
  Demux2/2 -> Mux1/2  "pe_est_[k]"
  Demux2/3 -> Mux1/3  "ph_est_[k]"
  Demux2/4 -> Mux1/4  "vn_est_[k]"
  Demux2/6 -> Add1/2  "vh_est_[k]"
  Demux2/5 -> Mux1/5  "ve_est_[k]"
  x_est_[k-1/k-1]/1 -> Demux2/1
  delta_[k]/1 -> Add1/1

== system NavigationObserver_4/Navigation Observer/EKF/K[k] (navigation)/Jacobian F/delta_vn ==
  x_est_[k-1/k-1] : Inport
  delta_[k] : Inport  Port=2
  Add : Sum
  Demux2 : Demux  Outputs=6
  Mux1 : Mux  Inputs=6
  x_est_[k-1/k-1]+delta_vn : Outport
  wires:
  Add/1 -> Mux1/4
  Mux1/1 -> x_est_[k-1/k-1]+delta_vn/1
  Demux2/1 -> Mux1/1  "pn_est_[k]"
  Demux2/2 -> Mux1/2  "pe_est_[k]"
  Demux2/3 -> Mux1/3  "ph_est_[k]"
  Demux2/4 -> Add/2  "vn_est_[k]"
  Demux2/6 -> Mux1/6  "vh_est_[k]"
  Demux2/5 -> Mux1/5  "ve_est_[k]"
  x_est_[k-1/k-1]/1 -> Demux2/1
  delta_[k]/1 -> Add/1

== system NavigationObserver_4/Navigation Observer/EKF/K[k] (navigation)/Jacobian F/f_(x_est_[k],u_[k]) ==
  u_[k-1] : Inport
  x_est_[k-1/k-1] : Inport  Port=2
  f(x_est_[k],u_[k]) : Subsystem
  f_(x_est_[k],u_[k]) : Outport
  wires:
  f(x_est_[k],u_[k])/1(f_(x_est_[k],u_[k])) -> f_(x_est_[k],u_[k])/1
  x_est_[k-1/k-1]/1 -> f(x_est_[k],u_[k])/1(x_est [k])
  u_[k-1]/1 -> f(x_est_[k],u_[k])/2(u_[k])

== system NavigationObserver_4/Navigation Observer/EKF/K[k] (navigation)/Jacobian F/f_(x_est_[k],u_[k])+delta_pe ==
  u_[k-1] : Inport
  x_est_[k-1/k-1] : Inport  Port=2
  f(x_est_[k],u_[k]) : Subsystem
  f_(x_est_[k],u_[k]) : Outport
  wires:
  f(x_est_[k],u_[k])/1(f_(x_est_[k],u_[k])) -> f_(x_est_[k],u_[k])/1
  x_est_[k-1/k-1]/1 -> f(x_est_[k],u_[k])/1(x_est [k])
  u_[k-1]/1 -> f(x_est_[k],u_[k])/2(u_[k])

== system NavigationObserver_4/Navigation Observer/EKF/K[k] (navigation)/Jacobian F/f_(x_est_[k],u_[k])+delta_ph ==
  u_[k-1] : Inport
  x_est_[k-1/k-1] : Inport  Port=2
  f(x_est_[k],u_[k]) : Subsystem
  f_(x_est_[k],u_[k]) : Outport
  wires:
  f(x_est_[k],u_[k])/1(f_(x_est_[k],u_[k])) -> f_(x_est_[k],u_[k])/1
  x_est_[k-1/k-1]/1 -> f(x_est_[k],u_[k])/1(x_est [k])
  u_[k-1]/1 -> f(x_est_[k],u_[k])/2(u_[k])

== system NavigationObserver_4/Navigation Observer/EKF/K[k] (navigation)/Jacobian F/f_(x_est_[k],u_[k])+delta_pn ==
  u_[k-1] : Inport
  x_est_[k-1/k-1] : Inport  Port=2
  f(x_est_[k],u_[k]) : Subsystem
  f_(x_est_[k],u_[k]) : Outport
  wires:
  f(x_est_[k],u_[k])/1(f_(x_est_[k],u_[k])) -> f_(x_est_[k],u_[k])/1
  x_est_[k-1/k-1]/1 -> f(x_est_[k],u_[k])/1(x_est [k])
  u_[k-1]/1 -> f(x_est_[k],u_[k])/2(u_[k])

== system NavigationObserver_4/Navigation Observer/EKF/K[k] (navigation)/Jacobian F/f_(x_est_[k],u_[k])+delta_ve ==
  u_[k-1] : Inport
  x_est_[k-1/k-1] : Inport  Port=2
  f(x_est_[k],u_[k]) : Subsystem
  f_(x_est_[k],u_[k]) : Outport
  wires:
  f(x_est_[k],u_[k])/1(f_(x_est_[k],u_[k])) -> f_(x_est_[k],u_[k])/1
  x_est_[k-1/k-1]/1 -> f(x_est_[k],u_[k])/1(x_est [k])
  u_[k-1]/1 -> f(x_est_[k],u_[k])/2(u_[k])

== system NavigationObserver_4/Navigation Observer/EKF/K[k] (navigation)/Jacobian F/f_(x_est_[k],u_[k])+delta_vh ==
  u_[k-1] : Inport
  x_est_[k-1/k-1] : Inport  Port=2
  f(x_est_[k],u_[k]) : Subsystem
  f_(x_est_[k],u_[k]) : Outport
  wires:
  f(x_est_[k],u_[k])/1(f_(x_est_[k],u_[k])) -> f_(x_est_[k],u_[k])/1
  x_est_[k-1/k-1]/1 -> f(x_est_[k],u_[k])/1(x_est [k])
  u_[k-1]/1 -> f(x_est_[k],u_[k])/2(u_[k])

== system NavigationObserver_4/Navigation Observer/EKF/K[k] (navigation)/Jacobian F/f_(x_est_[k],u_[k])+delta_vn ==
  u_[k-1] : Inport
  x_est_[k-1/k-1] : Inport  Port=2
  f(x_est_[k],u_[k]) : Subsystem
  f_(x_est_[k],u_[k]) : Outport
  wires:
  f(x_est_[k],u_[k])/1(f_(x_est_[k],u_[k])) -> f_(x_est_[k],u_[k])/1
  x_est_[k-1/k-1]/1 -> f(x_est_[k],u_[k])/1(x_est [k])
  u_[k-1]/1 -> f(x_est_[k],u_[k])/2(u_[k])

== system NavigationObserver_4/Navigation Observer/EKF/x_est_[k/k-1]/f(x_est_[k],u_[k])/f(ve_est_[k];u) ==
  note: ax [ft/sec2]
  note: ay [ft/sec2]
  note: az [ft/sec2]
  note: theta [rad]
  note: phi [rad]
  note: psi [rad]
  Accelerometer Meas : Inport
  "phi, theta, psi" : Inport  Port=2
  Add1 : Sum
  Add2 : Sum  Inputs=+++
  Add3 : Sum  Inputs=-+
  Demux1 : Demux  Outputs=3
  Demux2 : Demux  Outputs=3
  Divide{1,4,6..7} (4 alike) : Product  Inputs=**
  Divide2 : Product  Inputs=***
  Divide3 : Product  Inputs=***
  Divide5 : Product  Inputs=***
  Trigonometric Function : Trigonometry
  Trigonometric Function1 : Trigonometry  Operator=cos
  Trigonometric Function2 : Trigonometry
  Trigonometric Function3 : Trigonometry
  Trigonometric Function4 : Trigonometry  Operator=cos
  Trigonometric Function5 : Trigonometry  Operator=cos
  f(ve_est_[k];u) : Outport
  wires:
  Demux2/3 -> Trigonometric Function3/1, Trigonometric Function4/1
  Demux2/2 -> Trigonometric Function2/1, Trigonometric Function1/1
  Demux2/1 -> Trigonometric Function/1, Trigonometric Function5/1
  Demux1/2 -> Divide1/2
  Demux1/3 -> Divide7/2
  Trigonometric Function/1 -> Divide6/1, Divide2/2
  Trigonometric Function2/1 -> Divide5/1, Divide2/1
  Trigonometric Function4/1 -> Divide6/2, Divide4/2
  Trigonometric Function5/1 -> Divide5/2, Divide4/1
  Trigonometric Function3/1 -> Divide5/3, Divide2/3, Divide3/3
  Divide7/1 -> Add2/3
  Add3/1 -> Divide7/1
  Divide5/1 -> Add3/2
  Divide6/1 -> Add3/1
  Divide1/1 -> Add2/2
  Divide3/1 -> Add2/1
  Divide2/1 -> Add1/2
  Divide4/1 -> Add1/1
  Add1/1 -> Divide1/1
  Trigonometric Function1/1 -> Divide3/2
  Demux1/1 -> Divide3/1
  Add2/1 -> f(ve_est_[k];u)/1
  Accelerometer Meas/1 -> Demux1/1
  "phi, theta, psi"/1 -> Demux2/1

== system NavigationObserver_4/Navigation Observer/EKF/x_est_[k/k-1]/f(x_est_[k],u_[k])/f(vh_est_[k];u) ==
  note: ax [ft/sec2]
  note: ay [ft/sec2]
  note: az [ft/sec2]
  note: theta [rad]
  note: phi [rad]
  Accelerometer Meas : Inport
  "phi, theta, psi" : Inport  Port=2
  Add1 : Sum  Inputs=+--
  Demux1 : Demux  Outputs=3
  Demux2 : Demux  Outputs=3
  Divide1 : Product  Inputs=***
  Divide2 : Product  Inputs=**
  Divide3 : Product  Inputs=***
  Sum : Sum  Inputs=|+-  SampleTime=dt
  Terminator2 : Terminator
  Trigonometric Function : Trigonometry
  Trigonometric Function1 : Trigonometry  Operator=cos
  Trigonometric Function2 : Trigonometry
  Trigonometric Function4 : Trigonometry  Operator=cos
  Trigonometric Function5 : Trigonometry  Operator=cos
  gravity : Constant  Value=g
  f(vh_est_[k];u) : Outport
  wires:
  Demux2/1 -> Trigonometric Function4/1, Trigonometric Function2/1
  Demux2/2 -> Trigonometric Function5/1, Trigonometric Function1/1, Trigonometric Function/1
  Divide1/1 -> Add1/3
  Demux1/3 -> Divide1/3
  Trigonometric Function5/1 -> Divide1/2
  Trigonometric Function4/1 -> Divide1/1
  Divide2/1 -> Add1/1
  Divide3/1 -> Add1/2
  Demux1/2 -> Divide3/3
  Trigonometric Function2/1 -> Divide3/2
  Trigonometric Function1/1 -> Divide3/1
  Trigonometric Function/1 -> Divide2/2
  Demux1/1 -> Divide2/1
  Accelerometer Meas/1 -> Demux1/1
  "phi, theta, psi"/1 -> Demux2/1
  Demux2/3 -> Terminator2/1
  Add1/1 -> Sum/1
  Sum/1 -> f(vh_est_[k];u)/1
  gravity/1 -> Sum/2

== system NavigationObserver_4/Navigation Observer/EKF/x_est_[k/k-1]/f(x_est_[k],u_[k])/f(vn_est_[k];u) ==
  note: ax [ft/sec2]
  note: ay [ft/sec2]
  note: az [ft/sec2]
  note: theta [rad]
  note: phi [rad]
  note: psi [rad]
  Accelerometer Meas : Inport
  "phi, theta, psi" : Inport  Port=2
  Add1 : Sum  Inputs=-+
  Add2 : Sum  Inputs=+++
  Add3 : Sum
  Demux1 : Demux  Outputs=3
  Demux2 : Demux  Outputs=3
  Divide{1,4,6..7} (4 alike) : Product  Inputs=**
  Divide2 : Product  Inputs=***
  Divide3 : Product  Inputs=***
  Divide5 : Product  Inputs=***
  Trigonometric Function : Trigonometry
  Trigonometric Function1 : Trigonometry  Operator=cos
  Trigonometric Function2 : Trigonometry
  Trigonometric Function3 : Trigonometry
  Trigonometric Function4 : Trigonometry  Operator=cos
  Trigonometric Function5 : Trigonometry  Operator=cos
  f(vn_est_[k];u) : Outport
  wires:
  "phi, theta, psi"/1 -> Demux2/1
  Divide7/1 -> Add2/3
  Add3/1 -> Divide7/1
  Divide5/1 -> Add3/2
  Divide6/1 -> Add3/1
  Divide1/1 -> Add2/2
  Divide3/1 -> Add2/1
  Trigonometric Function/1 -> Divide6/1, Divide2/2
  Trigonometric Function2/1 -> Divide5/1, Divide2/1
  Trigonometric Function3/1 -> Divide6/2, Divide4/2
  Trigonometric Function5/1 -> Divide5/2, Divide4/1
  Divide2/1 -> Add1/2
  Divide4/1 -> Add1/1
  Add1/1 -> Divide1/1
  Trigonometric Function4/1 -> Divide5/3, Divide2/3, Divide3/3
  Trigonometric Function1/1 -> Divide3/2
  Demux2/3 -> Trigonometric Function3/1, Trigonometric Function4/1
  Demux2/1 -> Trigonometric Function/1, Trigonometric Function5/1
  Demux2/2 -> Trigonometric Function2/1, Trigonometric Function1/1
  Add2/1 -> f(vn_est_[k];u)/1
  Demux1/3 -> Divide7/2
  Demux1/2 -> Divide1/2
  Demux1/1 -> Divide3/1
  Accelerometer Meas/1 -> Demux1/1

== system NavigationObserver_4/Navigation Observer/EKF/x_est_[k/k-1]/f(x_est_[k],u_[k])/f_pe(x_est_[k],u[k]) ==
  Gain : Gain
  f_pe(x_est_[k],u[k]) : Outport
  wires:
  [ve_o] -> Gain/1
  Gain/1 -> f_pe(x_est_[k],u[k])/1

== system NavigationObserver_4/Navigation Observer/EKF/x_est_[k/k-1]/f(x_est_[k],u_[k])/f_ph(x_est_[k],u[k]) ==
  Gain : Gain
  f_ph(x_est_[k],u[k]) : Outport
  wires:
  [vh_o] -> Gain/1
  Gain/1 -> f_ph(x_est_[k],u[k])/1

== system NavigationObserver_4/Navigation Observer/EKF/x_est_[k/k-1]/f(x_est_[k],u_[k])/f_pn(x_est_[k],u[k]) ==
  Gain : Gain
  f_pn(x_est_[k],u[k]) : Outport
  wires:
  [vn_o] -> Gain/1
  Gain/1 -> f_pn(x_est_[k],u[k])/1

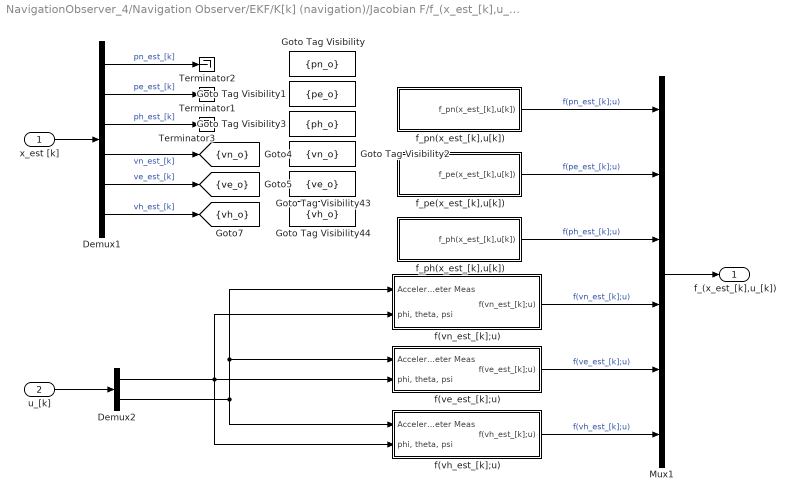
== system NavigationObserver_4/Navigation Observer/EKF/K[k] (navigation)/Jacobian F/f_(x_est_[k],u_[k])/f(x_est_[k],u_[k]) ==
  x_est [k] : Inport
  u_[k] : Inport  Port=2
  Demux1 : Demux  Outputs=6
  Demux2 : Demux  Outputs=2
  Goto Tag Visibility : GotoTagVisibility  GotoTag=pn_o
  Goto Tag Visibility1 : GotoTagVisibility  GotoTag=pe_o
  Goto Tag Visibility2 : GotoTagVisibility  GotoTag=vn_o
  Goto Tag Visibility3 : GotoTagVisibility  GotoTag=ph_o
  Goto Tag Visibility43 : GotoTagVisibility  GotoTag=ve_o
  Goto Tag Visibility44 : GotoTagVisibility  GotoTag=vh_o
  Mux1 : Mux  Inputs=6
  Terminator1 : Terminator
  Terminator2 : Terminator
  Terminator3 : Terminator
  f(ve_est_[k];u) : Subsystem
  f(vh_est_[k];u) : Subsystem
  f(vn_est_[k];u) : Subsystem
  f_pe(x_est_[k],u[k]) : Subsystem
  f_ph(x_est_[k],u[k]) : Subsystem
  f_pn(x_est_[k],u[k]) : Subsystem
  f_(x_est_[k],u_[k]) : Outport
  tag scope: ve_o=scoped, vh_o=scoped, vn_o=scoped
  wires:
  Demux2/2 -> f(vh_est_[k];u)/1(Accelerometer Meas), f(ve_est_[k];u)/1(Accelerometer Meas), f(vn_est_[k];u)/1(Accelerometer Meas)
  Demux2/1 -> f(vn_est_[k];u)/2("phi, theta, psi"), f(vh_est_[k];u)/2("phi, theta, psi"), f(ve_est_[k];u)/2("phi, theta, psi")
  u_[k]/1 -> Demux2/1
  f_pe(x_est_[k],u[k])/1(f_pe(x_est_[k],u[k])) -> Mux1/2  "f(pe_est_[k];u)"
  f_pn(x_est_[k],u[k])/1(f_pn(x_est_[k],u[k])) -> Mux1/1  "f(pn_est_[k];u)"
  f_ph(x_est_[k],u[k])/1(f_ph(x_est_[k],u[k])) -> Mux1/3  "f(ph_est_[k];u)"
  f(vn_est_[k];u)/1(f(vn_est_[k];u)) -> Mux1/4  "f(vn_est_[k];u)"
  f(ve_est_[k];u)/1(f(ve_est_[k];u)) -> Mux1/5  "f(ve_est_[k];u)"
  Mux1/1 -> f_(x_est_[k],u_[k])/1
  f(vh_est_[k];u)/1(f(vh_est_[k];u)) -> Mux1/6  "f(vh_est_[k];u)"
  Demux1/5 -> [ve_o]  "ve_est_[k]"
  x_est [k]/1 -> Demux1/1
  Demux1/6 -> [vh_o]  "vh_est_[k]"
  Demux1/4 -> [vn_o]  "vn_est_[k]"
  Demux1/3 -> Terminator3/1  "ph_est_[k]"
  Demux1/2 -> Terminator1/1  "pe_est_[k]"
  Demux1/1 -> Terminator2/1  "pn_est_[k]"

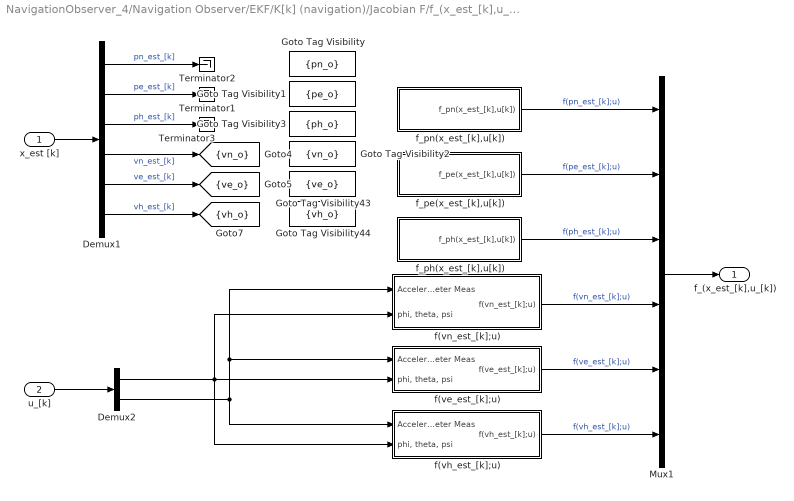
== system NavigationObserver_4/Navigation Observer/EKF/K[k] (navigation)/Jacobian F/f_(x_est_[k],u_[k])+delta_pe/f(x_est_[k],u_[k]) ==
  x_est [k] : Inport
  u_[k] : Inport  Port=2
  Demux1 : Demux  Outputs=6
  Demux2 : Demux  Outputs=2
  Goto Tag Visibility : GotoTagVisibility  GotoTag=pn_o
  Goto Tag Visibility1 : GotoTagVisibility  GotoTag=pe_o
  Goto Tag Visibility2 : GotoTagVisibility  GotoTag=vn_o
  Goto Tag Visibility3 : GotoTagVisibility  GotoTag=ph_o
  Goto Tag Visibility43 : GotoTagVisibility  GotoTag=ve_o
  Goto Tag Visibility44 : GotoTagVisibility  GotoTag=vh_o
  Mux1 : Mux  Inputs=6
  Terminator1 : Terminator
  Terminator2 : Terminator
  Terminator3 : Terminator
  f(ve_est_[k];u) : Subsystem
  f(vh_est_[k];u) : Subsystem
  f(vn_est_[k];u) : Subsystem
  f_pe(x_est_[k],u[k]) : Subsystem
  f_ph(x_est_[k],u[k]) : Subsystem
  f_pn(x_est_[k],u[k]) : Subsystem
  f_(x_est_[k],u_[k]) : Outport
  tag scope: ve_o=scoped, vh_o=scoped, vn_o=scoped
  wires:
  Demux2/2 -> f(vh_est_[k];u)/1(Accelerometer Meas), f(ve_est_[k];u)/1(Accelerometer Meas), f(vn_est_[k];u)/1(Accelerometer Meas)
  Demux2/1 -> f(vn_est_[k];u)/2("phi, theta, psi"), f(vh_est_[k];u)/2("phi, theta, psi"), f(ve_est_[k];u)/2("phi, theta, psi")
  u_[k]/1 -> Demux2/1
  f_pe(x_est_[k],u[k])/1(f_pe(x_est_[k],u[k])) -> Mux1/2  "f(pe_est_[k];u)"
  f_pn(x_est_[k],u[k])/1(f_pn(x_est_[k],u[k])) -> Mux1/1  "f(pn_est_[k];u)"
  f_ph(x_est_[k],u[k])/1(f_ph(x_est_[k],u[k])) -> Mux1/3  "f(ph_est_[k];u)"
  f(vn_est_[k];u)/1(f(vn_est_[k];u)) -> Mux1/4  "f(vn_est_[k];u)"
  f(ve_est_[k];u)/1(f(ve_est_[k];u)) -> Mux1/5  "f(ve_est_[k];u)"
  Mux1/1 -> f_(x_est_[k],u_[k])/1
  f(vh_est_[k];u)/1(f(vh_est_[k];u)) -> Mux1/6  "f(vh_est_[k];u)"
  Demux1/5 -> [ve_o]  "ve_est_[k]"
  x_est [k]/1 -> Demux1/1
  Demux1/6 -> [vh_o]  "vh_est_[k]"
  Demux1/4 -> [vn_o]  "vn_est_[k]"
  Demux1/3 -> Terminator3/1  "ph_est_[k]"
  Demux1/2 -> Terminator1/1  "pe_est_[k]"
  Demux1/1 -> Terminator2/1  "pn_est_[k]"

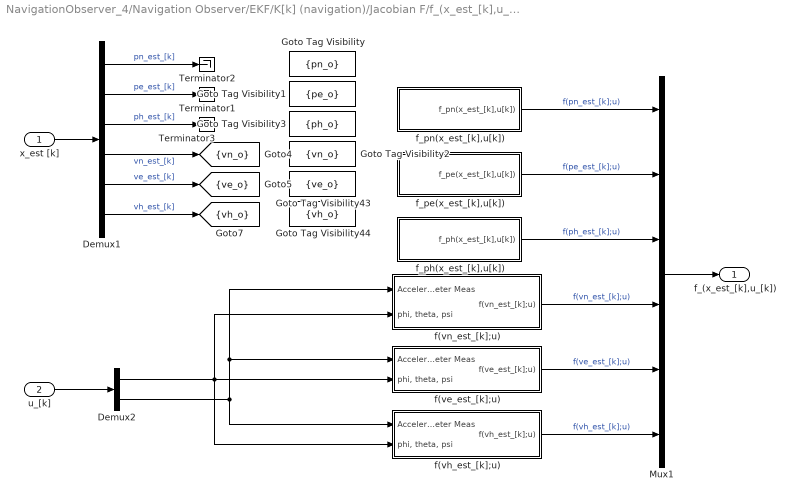
== system NavigationObserver_4/Navigation Observer/EKF/K[k] (navigation)/Jacobian F/f_(x_est_[k],u_[k])+delta_ph/f(x_est_[k],u_[k]) ==
  x_est [k] : Inport
  u_[k] : Inport  Port=2
  Demux1 : Demux  Outputs=6
  Demux2 : Demux  Outputs=2
  Goto Tag Visibility : GotoTagVisibility  GotoTag=pn_o
  Goto Tag Visibility1 : GotoTagVisibility  GotoTag=pe_o
  Goto Tag Visibility2 : GotoTagVisibility  GotoTag=vn_o
  Goto Tag Visibility3 : GotoTagVisibility  GotoTag=ph_o
  Goto Tag Visibility43 : GotoTagVisibility  GotoTag=ve_o
  Goto Tag Visibility44 : GotoTagVisibility  GotoTag=vh_o
  Mux1 : Mux  Inputs=6
  Terminator1 : Terminator
  Terminator2 : Terminator
  Terminator3 : Terminator
  f(ve_est_[k];u) : Subsystem
  f(vh_est_[k];u) : Subsystem
  f(vn_est_[k];u) : Subsystem
  f_pe(x_est_[k],u[k]) : Subsystem
  f_ph(x_est_[k],u[k]) : Subsystem
  f_pn(x_est_[k],u[k]) : Subsystem
  f_(x_est_[k],u_[k]) : Outport
  tag scope: ve_o=scoped, vh_o=scoped, vn_o=scoped
  wires:
  Demux2/2 -> f(vh_est_[k];u)/1(Accelerometer Meas), f(ve_est_[k];u)/1(Accelerometer Meas), f(vn_est_[k];u)/1(Accelerometer Meas)
  Demux2/1 -> f(vn_est_[k];u)/2("phi, theta, psi"), f(vh_est_[k];u)/2("phi, theta, psi"), f(ve_est_[k];u)/2("phi, theta, psi")
  u_[k]/1 -> Demux2/1
  f_pe(x_est_[k],u[k])/1(f_pe(x_est_[k],u[k])) -> Mux1/2  "f(pe_est_[k];u)"
  f_pn(x_est_[k],u[k])/1(f_pn(x_est_[k],u[k])) -> Mux1/1  "f(pn_est_[k];u)"
  f_ph(x_est_[k],u[k])/1(f_ph(x_est_[k],u[k])) -> Mux1/3  "f(ph_est_[k];u)"
  f(vn_est_[k];u)/1(f(vn_est_[k];u)) -> Mux1/4  "f(vn_est_[k];u)"
  f(ve_est_[k];u)/1(f(ve_est_[k];u)) -> Mux1/5  "f(ve_est_[k];u)"
  Mux1/1 -> f_(x_est_[k],u_[k])/1
  f(vh_est_[k];u)/1(f(vh_est_[k];u)) -> Mux1/6  "f(vh_est_[k];u)"
  Demux1/5 -> [ve_o]  "ve_est_[k]"
  x_est [k]/1 -> Demux1/1
  Demux1/6 -> [vh_o]  "vh_est_[k]"
  Demux1/4 -> [vn_o]  "vn_est_[k]"
  Demux1/3 -> Terminator3/1  "ph_est_[k]"
  Demux1/2 -> Terminator1/1  "pe_est_[k]"
  Demux1/1 -> Terminator2/1  "pn_est_[k]"

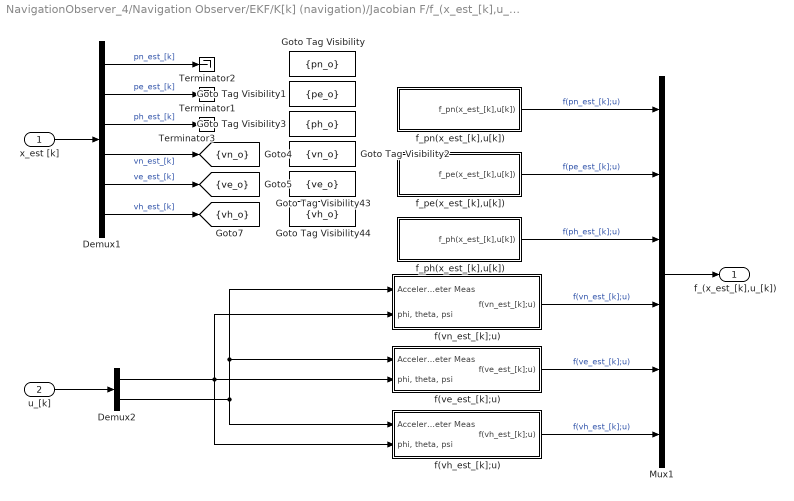
== system NavigationObserver_4/Navigation Observer/EKF/K[k] (navigation)/Jacobian F/f_(x_est_[k],u_[k])+delta_pn/f(x_est_[k],u_[k]) ==
  x_est [k] : Inport
  u_[k] : Inport  Port=2
  Demux1 : Demux  Outputs=6
  Demux2 : Demux  Outputs=2
  Goto Tag Visibility : GotoTagVisibility  GotoTag=pn_o
  Goto Tag Visibility1 : GotoTagVisibility  GotoTag=pe_o
  Goto Tag Visibility2 : GotoTagVisibility  GotoTag=vn_o
  Goto Tag Visibility3 : GotoTagVisibility  GotoTag=ph_o
  Goto Tag Visibility43 : GotoTagVisibility  GotoTag=ve_o
  Goto Tag Visibility44 : GotoTagVisibility  GotoTag=vh_o
  Mux1 : Mux  Inputs=6
  Terminator1 : Terminator
  Terminator2 : Terminator
  Terminator3 : Terminator
  f(ve_est_[k];u) : Subsystem
  f(vh_est_[k];u) : Subsystem
  f(vn_est_[k];u) : Subsystem
  f_pe(x_est_[k],u[k]) : Subsystem
  f_ph(x_est_[k],u[k]) : Subsystem
  f_pn(x_est_[k],u[k]) : Subsystem
  f_(x_est_[k],u_[k]) : Outport
  tag scope: ve_o=scoped, vh_o=scoped, vn_o=scoped
  wires:
  Demux2/2 -> f(vh_est_[k];u)/1(Accelerometer Meas), f(ve_est_[k];u)/1(Accelerometer Meas), f(vn_est_[k];u)/1(Accelerometer Meas)
  Demux2/1 -> f(vn_est_[k];u)/2("phi, theta, psi"), f(vh_est_[k];u)/2("phi, theta, psi"), f(ve_est_[k];u)/2("phi, theta, psi")
  u_[k]/1 -> Demux2/1
  f_pe(x_est_[k],u[k])/1(f_pe(x_est_[k],u[k])) -> Mux1/2  "f(pe_est_[k];u)"
  f_pn(x_est_[k],u[k])/1(f_pn(x_est_[k],u[k])) -> Mux1/1  "f(pn_est_[k];u)"
  f_ph(x_est_[k],u[k])/1(f_ph(x_est_[k],u[k])) -> Mux1/3  "f(ph_est_[k];u)"
  f(vn_est_[k];u)/1(f(vn_est_[k];u)) -> Mux1/4  "f(vn_est_[k];u)"
  f(ve_est_[k];u)/1(f(ve_est_[k];u)) -> Mux1/5  "f(ve_est_[k];u)"
  Mux1/1 -> f_(x_est_[k],u_[k])/1
  f(vh_est_[k];u)/1(f(vh_est_[k];u)) -> Mux1/6  "f(vh_est_[k];u)"
  Demux1/5 -> [ve_o]  "ve_est_[k]"
  x_est [k]/1 -> Demux1/1
  Demux1/6 -> [vh_o]  "vh_est_[k]"
  Demux1/4 -> [vn_o]  "vn_est_[k]"
  Demux1/3 -> Terminator3/1  "ph_est_[k]"
  Demux1/2 -> Terminator1/1  "pe_est_[k]"
  Demux1/1 -> Terminator2/1  "pn_est_[k]"
